simulink model "untitled5"  (Simulink 9.3)
settings: Solver=VariableStepAuto  StartTime=0.0  StopTime=25  RelTol=1e-3
libraries: Solver_SF x1, fuzblock x1
settings Model: Creator=lenovo  LastModifiedBy=lenovo
settings SolverCC: ZeroCrossAlgorithm=Adaptive
settings DataIOCC: SaveFormat=Dataset  SignalLoggingSaveFormat=Dataset  ReturnWorkspaceOutputs=on
settings OptimizationCC: LifeSpan=auto
settings DebuggingCC: UnderspecifiedInitializationDetection=Simplified  MergeDetectMultiDrivingBlocksExec=error  IgnoredZcDiagnostic=none  FcnCallInpInsideContextMsg=error  SFUnexpectedBacktrackingDiag=error  SFNoUnconditionalDefaultTransitionDiag=error  SFExecutionAtInitializationDiag=warning  ArithmeticOperatorsInVariantConditions=error
settings HardwareCC: ProdBitPerPointer=64  ProdBitPerSizeT=64  ProdBitPerPtrDiffT=64  ProdLargestAtomicFloat=Float  ProdIntDivRoundTo=Zero  ProdEndianess=LittleEndian  ProdWordSize=64  ProdHWDeviceType=Intel->x86-64 (Windows64)
settings ModelReferenceCC: PropagateSignalLabelsOutOfModel=on
settings SFSimCC: SimUseLocalCustomCode=on
settings RTWCC: RTWUseLocalCustomCode=on
settings CodeAppCC: StateflowObjectComments=off
settings GRTTargetCC: TargetLangStandard=C99 (ISO)  CombineOutputUpdateFcns=on  GRTInterface=off
settings ConfigComp: CovMetricSettings=dwe  CovHtmlReporting=off  CovSaveCumulativeToWorkspaceVar=off  CovSaveSingleToWorkspaceVar=off  CovExternalEMLEnable=on

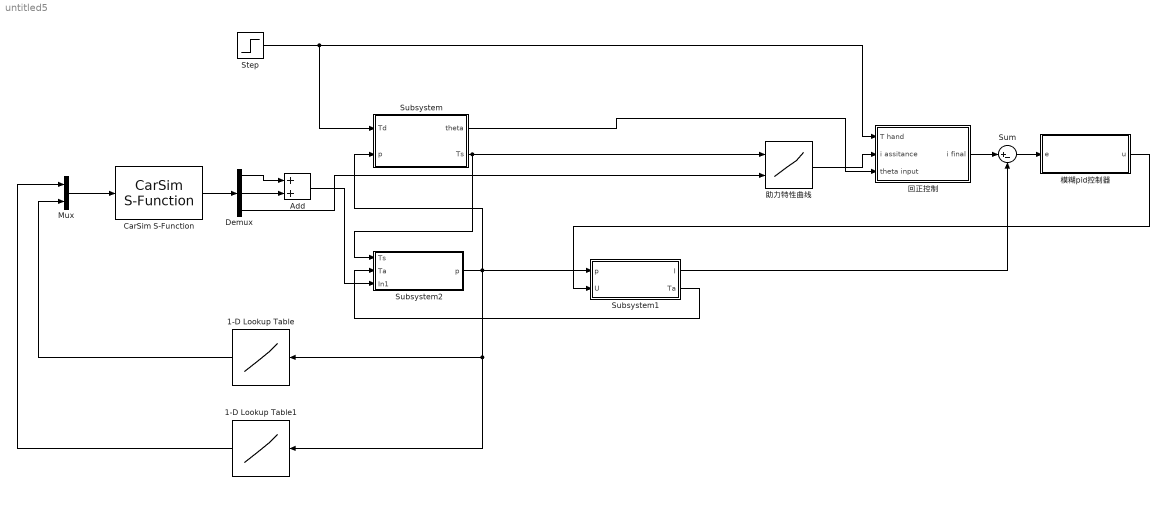
== system untitled5 ==
  1-D Lookup Table : Lookup_n-D  NumberOfTableDimensions=1  BreakpointsForDimension1=[0,5,10,15,20,25,30,35,40,45,50,55,60,65,70,75,80]  Table=[2,4,6,8,10,12,14,16,18,20,22,24,27,29,31,33,36]  InternalRulePriority=Speed  RndMeth=Simplest  InputSameDT=on
  1-D Lookup Table1 : Lookup_n-D  NumberOfTableDimensions=1  BreakpointsForDimension1=[0,5,10,15,20,25,30,35,40,45,50,55,60,65,70,75,80]  Table=[2,4,6,8,10,12,14,16,18,20,22,24,27,29,31,33,36]  InternalRulePriority=Speed  RndMeth=Simplest  InputSameDT=on
  Add : Sum
  CarSim S-Function : Solver_SF/CarSim S-Function  Priority=1  VehicleCode=i_i  SIMFILE=simfile
  Demux : Demux  Outputs=3
  Mux : Mux  Inputs=2
  Step : Step  SampleTime=0
  Subsystem : Subsystem
  Subsystem1 : Subsystem
  Subsystem2 : Subsystem
  Sum : Sum  Inputs=|+-
  助力特性曲线 : Lookup_n-D  BreakpointsForDimension1=[-16,-7.6,-1,0,1,7.6,16]  BreakpointsForDimension2=[0,10,20,30,40,60,70]  Table=reshape([-12.68,-12.68,0,0,0,12.68,12.68,-8.14,-8.14,0,0,0,8.14,8.14,-7.31,-7.31,0,0,0,7.31,7.31,-6.14,-6.14,0,0,0,6.14,6.14,-5.01,-5.01,0,0,0,5.01,5.01,-4.24,-4.24,0,0,0,4.24,4.24,-1.98,-1.98,0,0,0,1.98,1.98],7,7)  InternalRulePriority=Speed  RndMeth=Simplest  InputSameDT=on
  回正控制 : Subsystem
  模糊pid控制器 : Subsystem
  wires:
  Subsystem2/1(p) -> 1-D Lookup Table/1, 1-D Lookup Table1/1, Subsystem1/1(p), Subsystem/2(p)
  模糊pid控制器/1(u) -> Subsystem1/2("U ")
  Subsystem1/2(Ta) -> Subsystem2/2(Ta)
  Subsystem1/1(I) -> Sum/2
  Subsystem/1(theta) -> 回正控制/3("theta input ")
  Subsystem/2(Ts) -> Subsystem2/1(Ts), 助力特性曲线/1
  助力特性曲线/1 -> 回正控制/2(i assitance)
  回正控制/1(i final) -> Sum/1
  Sum/1 -> 模糊pid控制器/1("e ")
  CarSim S-Function/1 -> Demux/1
  Add/1 -> Subsystem2/3(In1)
  Demux/2 -> Add/2
  Demux/3 -> 助力特性曲线/2
  Demux/1 -> Add/1
  Step/1 -> 回正控制/1("T hand "), Subsystem/1(Td)
  Mux/1 -> CarSim S-Function/1
  1-D Lookup Table/1 -> Mux/2
  1-D Lookup Table1/1 -> Mux/1

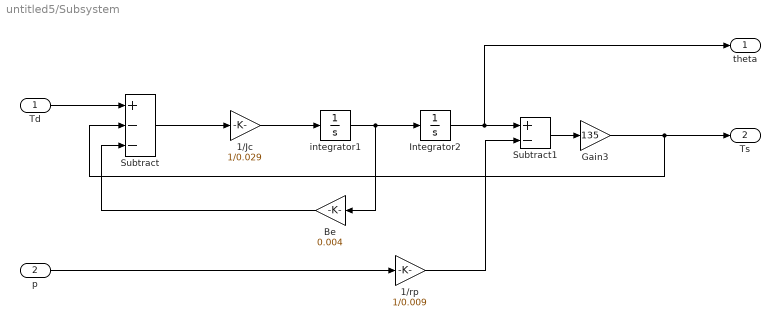
== system untitled5/Subsystem ==
  Td : Inport
  p : Inport  Port=2
  1/Jc : Gain  Gain=1/0.029
  1/rp : Gain  Gain=1/0.009
  Be : Gain  Gain=0.004
  Gain3 : Gain  Gain=135
  "Integrator2 " : Integrator
  Subtract : Sum  Inputs=+--
  Subtract1 : Sum  Inputs=+-
  "integrator1 " : Integrator
  theta : Outport
  Ts : Outport  Port=2
  wires:
  Be/1 -> Subtract/3
  1/rp/1 -> Subtract1/2
  p/1 -> 1/rp/1
  "Integrator2 "/1 -> theta/1, Subtract1/1
  "integrator1 "/1 -> "Integrator2 "/1, Be/1
  Subtract/1 -> 1/Jc/1
  Gain3/1 -> Subtract/2, Ts/1
  Subtract1/1 -> Gain3/1
  1/Jc/1 -> "integrator1 "/1
  Td/1 -> Subtract/1

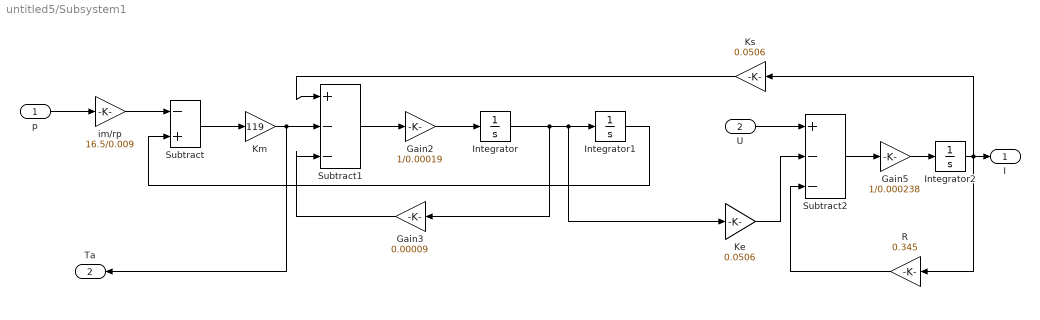
== system untitled5/Subsystem1 ==
  p : Inport
  "U " : Inport  Port=2
  Gain2 : Gain  Gain=1/0.00019
  Gain3 : Gain  Gain=0.00009
  Gain5 : Gain  Gain=1/0.000238
  Integrator : Integrator
  Integrator1 : Integrator
  Integrator2 : Integrator
  Ke : Gain  Gain=0.0506
  Km : Gain  Gain=119
  Ks : Gain  Gain=0.0506
  R : Gain  Gain=0.345
  Subtract : Sum  Inputs=-+
  Subtract1 : Sum  Inputs=+--
  Subtract2 : Sum  Inputs=+--
  im/rp : Gain  Gain=16.5/0.009
  I : Outport
  Ta : Outport  Port=2
  wires:
  Gain2/1 -> Integrator/1
  Gain5/1 -> Integrator2/1
  Ke/1 -> Subtract2/2
  Km/1 -> Ta/1, Subtract1/2
  Subtract2/1 -> Gain5/1
  Subtract1/1 -> Gain2/1
  Subtract/1 -> Km/1
  Integrator1/1 -> Subtract/2
  "U "/1 -> Subtract2/1
  Integrator2/1 -> R/1, Ks/1, I/1
  Gain3/1 -> Subtract1/3
  im/rp/1 -> Subtract/1
  R/1 -> Subtract2/3
  p/1 -> im/rp/1
  Integrator/1 -> Gain3/1, Ke/1, Integrator1/1
  Ks/1 -> Subtract1/1

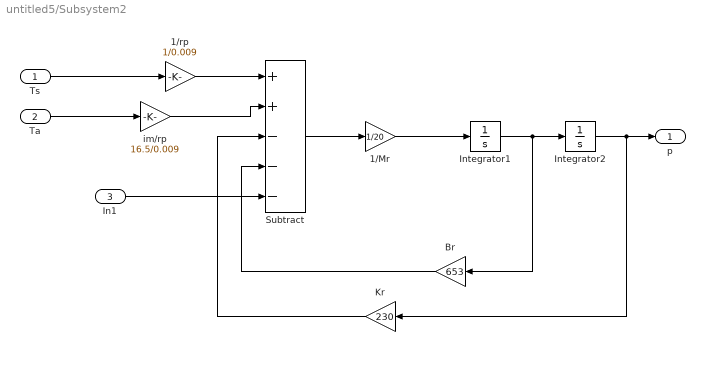
== system untitled5/Subsystem2 ==
  Ts : Inport
  Ta : Inport  Port=2
  In1 : Inport  Port=3
  1/Mr : Gain  Gain=1/20
  1/rp : Gain  Gain=1/0.009
  Br : Gain  Gain=653
  "Integrator1 " : Integrator
  "Integrator2 " : Integrator
  Kr : Gain  Gain=230
  Subtract : Sum  Inputs=++---
  im/rp : Gain  Gain=16.5/0.009
  p : Outport
  wires:
  im/rp/1 -> Subtract/2
  "Integrator1 "/1 -> Br/1, "Integrator2 "/1
  1/Mr/1 -> "Integrator1 "/1
  Ts/1 -> 1/rp/1
  Subtract/1 -> 1/Mr/1
  Kr/1 -> Subtract/3
  1/rp/1 -> Subtract/1
  Ta/1 -> im/rp/1
  Br/1 -> Subtract/4
  "Integrator2 "/1 -> Kr/1, p/1
  In1/1 -> Subtract/5

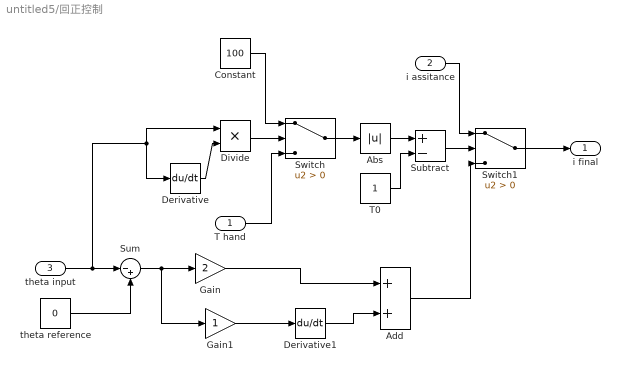
== system untitled5/回正控制 ==
  "T hand " : Inport
  i assitance : Inport  Port=2
  "theta input " : Inport  Port=3
  Abs : Abs
  Add : Sum
  Constant : Constant  Value=100
  Derivative : Derivative
  Derivative1 : Derivative
  Divide : Product  Inputs=**
  Gain : Gain  Gain=2
  Gain1 : Gain
  Subtract : Sum  Inputs=+-
  Sum : Sum  Inputs=|-+
  Switch : Switch  Criteria=u2 > Threshold
  Switch1 : Switch  Criteria=u2 > Threshold
  "T0 " : Constant
  theta reference : Constant  Value=0
  i final : Outport
  wires:
  Add/1 -> Switch1/3
  Derivative1/1 -> Add/2
  Derivative/1 -> Divide/2
  Gain1/1 -> Derivative1/1
  i assitance/1 -> Switch1/1
  Switch1/1 -> i final/1
  Abs/1 -> Subtract/1
  Divide/1 -> Switch/2
  Sum/1 -> Gain/1, Gain1/1
  Constant/1 -> Switch/1
  Switch/1 -> Abs/1
  "T0 "/1 -> Subtract/2
  "T hand "/1 -> Switch/3
  Gain/1 -> Add/1
  "theta input "/1 -> Sum/1, Divide/1, Derivative/1
  theta reference/1 -> Sum/2
  Subtract/1 -> Switch1/2

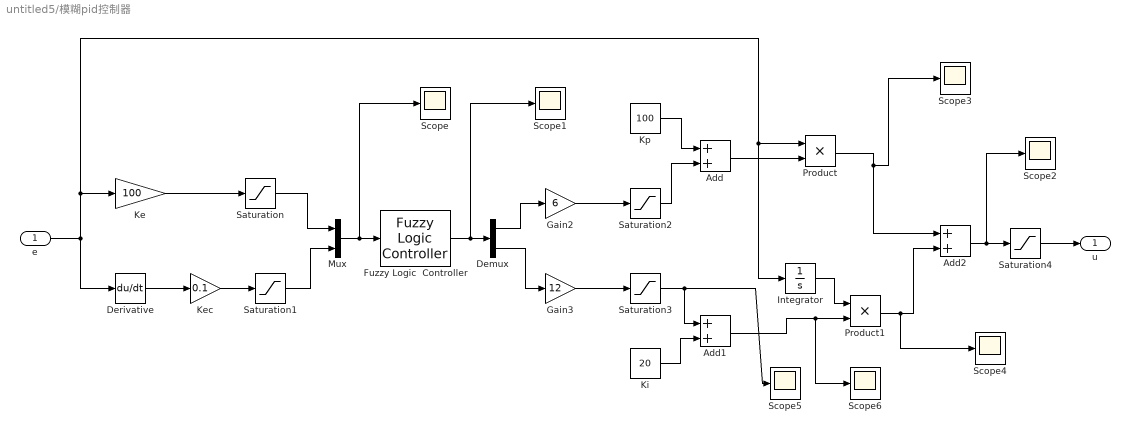
== system untitled5/模糊pid控制器 ==
  "e " : Inport
  Add : Sum
  Add1 : Sum
  Add2 : Sum
  Demux : Demux  Outputs=2
  Derivative : Derivative
  Fuzzy Logic  Controller : fuzblock/Fuzzy Logic  Controller  FIS='adptivefuzzypidcontrol.fis'  OutputSampleNumber=101  DataType=double  FuzzifiedInputs=off  RuleFiringStrengths=off  RuleOutputs=off  AggregatedOutputs=off  SimulateUsing=Interpreted execution  OutOfRangeInputValueMessage=warning  NoRuleFiredMessage=warning  EmptyOutputFuzzySetMessage=warning
  Gain2 : Gain  Gain=6
  Gain3 : Gain  Gain=12
  Integrator : Integrator
  Ke : Gain  Gain=100
  Kec : Gain  Gain=0.1
  Ki : Constant  Value=20
  Kp : Constant  Value=100
  Mux : Mux  Inputs=2
  Product : Product
  Product1 : Product
  Saturation{,1..3} (4 alike) : Saturate  UpperLimit=6  LowerLimit=-6
  Saturation4 : Saturate  UpperLimit=12  LowerLimit=-12
  Scope{,1..6} (7 alike) : Scope
  u : Outport
  wires:
  Add1/1 -> Scope6/1, Product1/2
  Saturation2/1 -> Add/2
  Kp/1 -> Add/1
  Saturation3/1 -> Scope5/1, Add1/1
  Integrator/1 -> Product1/1
  Add/1 -> Product/2
  Ke/1 -> Saturation/1
  Add2/1 -> Scope2/1, Saturation4/1
  Demux/2 -> Gain3/1
  Demux/1 -> Gain2/1
  Gain3/1 -> Saturation3/1
  Gain2/1 -> Saturation2/1
  Saturation1/1 -> Mux/2
  Fuzzy Logic  Controller/1 -> Scope1/1, Demux/1
  "e "/1 -> Derivative/1, Product/1, Integrator/1, Ke/1
  Product1/1 -> Scope4/1, Add2/2
  Product/1 -> Scope3/1, Add2/1
  Derivative/1 -> Kec/1
  Saturation/1 -> Mux/1
  Mux/1 -> Fuzzy Logic  Controller/1, Scope/1
  Ki/1 -> Add1/2
  Saturation4/1 -> u/1
  Kec/1 -> Saturation1/1
